simulink model "Boeing737Sample_updatedCopy"  (Simulink 8.2)
settings: Solver=ode45  StartTime=0.0  StopTime=100  RelTol=1e-3
InitFcn:
  | load('loss_coeff_mixing_junction.mat')
  | %load('defaultMSSN.mat')
  | load('SampleOutput.mat')
  | load('HydProp.mat')
  | load('HydraulicLoad.mat')
  | load('initavload.mat')
  | %load('mission_short.mat')
values from neighbouring files (symbols this model uses):
  avload =     [Benchmark_data1.mat]
  FuelBurn = [0 0 0 0 0 0 0 0 0 0 0 0 ... (18249 elements, 1x18249)]    [Benchmark_data1.mat]
undefined symbols (not defined in the file or in its folder): ailerons, B_737, elevator, F1, F2, HUGHES_TREITLER, landing_gear, PN_70147, rudder, thrust_rev
libraries: PowerFlowLib x91, simulink x19
(part 6 of 8)

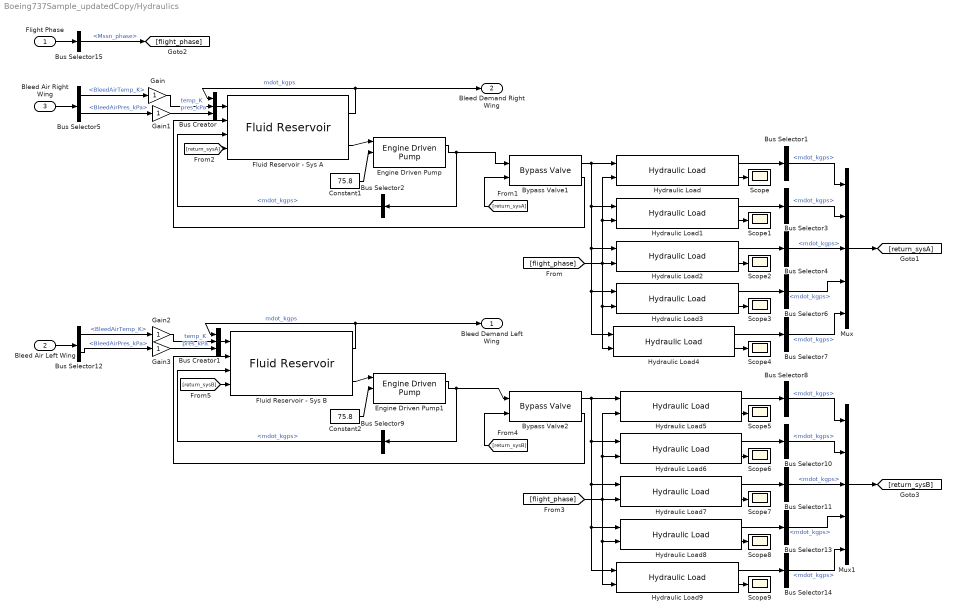
== system Boeing737Sample_updatedCopy/Hydraulics  ==
  Flight Phase : Inport
  Bleed Air Left Wing : Inport  Port=2
  Bleed Air Right Wing : Inport  Port=3
  Bus Creator : BusCreator  Inputs=3
  Bus Creator1 : BusCreator  Inputs=3
  Bus Selector{1..4,6..11,13..14} (12 alike) : BusSelector  OutputSignals=mdot_kgps
  Bus Selector12 : BusSelector  OutputSignals=Bleed.BleedAirTemp_K,Bleed.BleedAirPres_kPa
  Bus Selector15 : BusSelector  OutputSignals=Mssn_phase
  Bus Selector5 : BusSelector  OutputSignals=Bleed.BleedAirTemp_K,Bleed.BleedAirPres_kPa
  Bypass Valve1 : PowerFlowLib/Energy & Power Systems/Hydraulic/Bypass Valve
  Bypass Valve2 : PowerFlowLib/Energy & Power Systems/Hydraulic/Bypass Valve
  Constant1 : Constant  Value=75.8
  Constant2 : Constant  Value=75.8
  Engine Driven Pump : PowerFlowLib/Energy & Power Systems/Hydraulic/Engine Driven Pump  RPM=3750  disp=39  eta_mech=95  eta_v=85  nom_T=40  nom_w=393  nom_delP=20684
  Engine Driven Pump1 : PowerFlowLib/Energy & Power Systems/Hydraulic/Engine Driven Pump  RPM=3750  disp=39  eta_mech=95  eta_v=85  nom_T=40  nom_w=393  nom_delP=20684
  Fluid Reservoir - Sys A : PowerFlowLib/Energy & Power Systems/Hydraulic/Fluid Reservoir  res_vol=.25  bleed_flowrate=.05  pres_loss=1  T_init=300  P_init=1500  mass_init=30
  Fluid Reservoir - Sys B : PowerFlowLib/Energy & Power Systems/Hydraulic/Fluid Reservoir  res_vol=.25  bleed_flowrate=.05  pres_loss=1  T_init=300  P_init=1500  mass_init=30
  Gain{,1..3} (4 alike) : Gain
  Hydraulic Load : PowerFlowLib/Energy & Power Systems/Hydraulic/Hydraulic Load  fileslct=off  filename=HydraulicLoad.mat  filedir=C:\Users\mwillms4\Dropbox\School\Graduate\Research\PowerFlow Development\PowerFlow Summer 2013\PropertyTables\HydraulicLoad.mat  var_struct=HydraulicLoad  h_load=B_737 - rudder
  Hydraulic Load1 : PowerFlowLib/Energy & Power Systems/Hydraulic/Hydraulic Load  fileslct=off  filename=HydraulicLoad.mat  filedir=C:\Users\mwillms4\Dropbox\School\Graduate\Research\PowerFlow Development\PowerFlow Summer 2013\PropertyTables\HydraulicLoad.mat  var_struct=HydraulicLoad  h_load=B_737 - ailerons
  Hydraulic Load2 : PowerFlowLib/Energy & Power Systems/Hydraulic/Hydraulic Load  fileslct=off  filename=HydraulicLoad.mat  filedir=C:\Users\mwillms4\Dropbox\School\Graduate\Research\PowerFlow Development\PowerFlow Summer 2013\PropertyTables\HydraulicLoad.mat  var_struct=HydraulicLoad  h_load=B_737 - elevator
  Hydraulic Load3 : PowerFlowLib/Energy & Power Systems/Hydraulic/Hydraulic Load  fileslct=off  filename=HydraulicLoad.mat  filedir=C:\Users\mwillms4\Dropbox\School\Graduate\Research\PowerFlow Development\PowerFlow Summer 2013\PropertyTables\HydraulicLoad.mat  var_struct=HydraulicLoad  h_load=B_737 - landing_gear
  Hydraulic Load4 : PowerFlowLib/Energy & Power Systems/Hydraulic/Hydraulic Load  fileslct=off  filename=HydraulicLoad.mat  filedir=C:\Users\mwillms4\Dropbox\School\Graduate\Research\PowerFlow Development\PowerFlow Summer 2013\PropertyTables\HydraulicLoad.mat  var_struct=HydraulicLoad  h_load=B_737 - thrust_rev
  Hydraulic Load5 : PowerFlowLib/Energy & Power Systems/Hydraulic/Hydraulic Load  fileslct=off  filename=HydraulicLoad.mat  filedir=C:\Users\mwillms4\Dropbox\School\Graduate\Research\PowerFlow Development\PowerFlow Summer 2013\PropertyTables\HydraulicLoad.mat  var_struct=HydraulicLoad  h_load=B_737 - rudder
  Hydraulic Load6 : PowerFlowLib/Energy & Power Systems/Hydraulic/Hydraulic Load  fileslct=off  filename=HydraulicLoad.mat  filedir=C:\Users\mwillms4\Dropbox\School\Graduate\Research\PowerFlow Development\PowerFlow Summer 2013\PropertyTables\HydraulicLoad.mat  var_struct=HydraulicLoad  h_load=B_737 - ailerons
  Hydraulic Load7 : PowerFlowLib/Energy & Power Systems/Hydraulic/Hydraulic Load  fileslct=off  filename=HydraulicLoad.mat  filedir=C:\Users\mwillms4\Dropbox\School\Graduate\Research\PowerFlow Development\PowerFlow Summer 2013\PropertyTables\HydraulicLoad.mat  var_struct=HydraulicLoad  h_load=B_737 - elevator
  Hydraulic Load8 : PowerFlowLib/Energy & Power Systems/Hydraulic/Hydraulic Load  fileslct=off  filename=HydraulicLoad.mat  filedir=C:\Users\mwillms4\Dropbox\School\Graduate\Research\PowerFlow Development\PowerFlow Summer 2013\PropertyTables\HydraulicLoad.mat  var_struct=HydraulicLoad  h_load=B_737 - landing_gear
  Hydraulic Load9 : PowerFlowLib/Energy & Power Systems/Hydraulic/Hydraulic Load  fileslct=off  filename=HydraulicLoad.mat  filedir=C:\Users\mwillms4\Dropbox\School\Graduate\Research\PowerFlow Development\PowerFlow Summer 2013\PropertyTables\HydraulicLoad.mat  var_struct=HydraulicLoad  h_load=B_737 - thrust_rev
  Mux : Mux  Inputs=5
  Mux1 : Mux  Inputs=5
  Scope{,1..9} (10 alike) : Scope
      Scope1 settings: SaveName=ScopeData4
      Scope2 settings: YMin=0  YMax=55  SaveName=ScopeData5
      Scope3 settings: YMin=0  YMax=55
      Scope4 settings: YMin=0  YMax=55  SaveName=ScopeData2
      Scope5 settings: SaveName=ScopeData3
      Scope6 settings: SaveName=ScopeData6
      Scope7 settings: YMin=0  YMax=55  SaveName=ScopeData7
      Scope8 settings: YMin=0  YMax=55  SaveName=ScopeData8
      Scope9 settings: YMin=0  YMax=55  SaveName=ScopeData9
  Bleed Demand Left Wing : Outport
  Bleed Demand Right Wing : Outport  Port=2
  wires:
  Bus Creator/1 -> Fluid Reservoir - Sys A/1
  Bus Selector5/1 -> Gain/1  "<BleedAirTemp_K>"
  Bus Selector5/2 -> Gain1/1  "<BleedAirPres_kPa>"
  Hydraulic Load/1 -> Bus Selector1/1
  Fluid Reservoir - Sys A/2 -> Engine Driven Pump/1
  Engine Driven Pump/1 -> Bus Selector2/1, Bypass Valve1/1
  Bypass Valve1/1 -> Hydraulic Load3/1, Hydraulic Load4/1, Hydraulic Load2/1, Hydraulic Load1/1, Hydraulic Load/1
  Constant1/1 -> Engine Driven Pump/2
  Bus Selector2/1 -> Fluid Reservoir - Sys A/3  "<mdot_kgps>"
  Bypass Valve1/2 -> Fluid Reservoir - Sys A/2
  Hydraulic Load/2 -> Scope/1
  Fluid Reservoir - Sys A/1 -> Bus Creator/1, Bleed Demand Right Wing/1  "mdot_kgps"
  Hydraulic Load1/2 -> Scope1/1
  Hydraulic Load2/2 -> Scope2/1
  Hydraulic Load1/1 -> Bus Selector3/1
  Hydraulic Load2/1 -> Bus Selector4/1
  Bus Selector3/1 -> Mux/2  "<mdot_kgps>"
  Bus Selector1/1 -> Mux/1  "<mdot_kgps>"
  Bus Selector4/1 -> Mux/3  "<mdot_kgps>"
  Mux/1 -> [return_sysA]
  [return_sysA] -> Bypass Valve1/2
  [return_sysA] -> Fluid Reservoir - Sys A/4
  [flight_phase] -> Hydraulic Load/2, Hydraulic Load1/2, Hydraulic Load3/2, Hydraulic Load4/2, Hydraulic Load2/2
  Bleed Air Right Wing/1 -> Bus Selector5/1
  Hydraulic Load3/1 -> Bus Selector6/1
  Hydraulic Load4/1 -> Bus Selector7/1
  Hydraulic Load4/2 -> Scope4/1
  Hydraulic Load3/2 -> Scope3/1
  Bus Selector6/1 -> Mux/4  "<mdot_kgps>"
  Bus Selector7/1 -> Mux/5  "<mdot_kgps>"
  Bus Creator1/1 -> Fluid Reservoir - Sys B/1
  Bus Selector12/1 -> Gain2/1  "<BleedAirTemp_K>"
  Bus Selector12/2 -> Gain3/1  "<BleedAirPres_kPa>"
  Hydraulic Load5/1 -> Bus Selector8/1
  Fluid Reservoir - Sys B/2 -> Engine Driven Pump1/1
  Engine Driven Pump1/1 -> Bus Selector9/1, Bypass Valve2/1
  Bypass Valve2/1 -> Hydraulic Load9/1, Hydraulic Load8/1, Hydraulic Load7/1, Hydraulic Load6/1, Hydraulic Load5/1
  Constant2/1 -> Engine Driven Pump1/2
  Bus Selector9/1 -> Fluid Reservoir - Sys B/3  "<mdot_kgps>"
  Bypass Valve2/2 -> Fluid Reservoir - Sys B/2
  Hydraulic Load5/2 -> Scope5/1
  Fluid Reservoir - Sys B/1 -> Bus Creator1/1, Bleed Demand Left Wing/1  "mdot_kgps"
  Hydraulic Load6/2 -> Scope6/1
  Hydraulic Load7/2 -> Scope7/1
  Hydraulic Load6/1 -> Bus Selector10/1
  Hydraulic Load7/1 -> Bus Selector11/1
  Bus Selector10/1 -> Mux1/2  "<mdot_kgps>"
  Bus Selector8/1 -> Mux1/1  "<mdot_kgps>"
  Bus Selector11/1 -> Mux1/3  "<mdot_kgps>"
  Mux1/1 -> [return_sysB]
  [return_sysB] -> Bypass Valve2/2
  [return_sysB] -> Fluid Reservoir - Sys B/4
  [flight_phase] -> Hydraulic Load6/2, Hydraulic Load5/2, Hydraulic Load9/2, Hydraulic Load8/2, Hydraulic Load7/2
  Bleed Air Left Wing/1 -> Bus Selector12/1
  Hydraulic Load8/1 -> Bus Selector13/1
  Hydraulic Load9/1 -> Bus Selector14/1
  Hydraulic Load9/2 -> Scope9/1
  Hydraulic Load8/2 -> Scope8/1
  Bus Selector13/1 -> Mux1/4  "<mdot_kgps>"
  Bus Selector14/1 -> Mux1/5  "<mdot_kgps>"
  Flight Phase/1 -> Bus Selector15/1
  Bus Selector15/1 -> [flight_phase]  "<Mssn_phase>"
  Gain/1 -> Bus Creator/2  "temp_K"
  Gain1/1 -> Bus Creator/3  "pres_kPa"
  Gain2/1 -> Bus Creator1/2  "temp_K"
  Gain3/1 -> Bus Creator1/3  "pres_kPa"

== system Boeing737Sample_updatedCopy/PowerFlow Data Manager ==
  Data : Outport

== system Boeing737Sample_updatedCopy/ECS & FOS /Distributor valve ==
  Flow from Right Pack : Inport
  "Distribution ratio, R" : Inport  Port=2
  Bus Creator : BusCreator  Inputs=3
  Bus Creator1 : BusCreator  Inputs=3
  Bus Selector1 : BusSelector  OutputSignals=mdot_kgps,temp_K,pres_kPa
  M(1-R) : Sum  Inputs=+-
  Product : Product
  To cargo : Outport
  To Mix Junction : Outport  Port=2
  wires:
  Flow from Right Pack/1 -> Bus Selector1/1
  Bus Selector1/1 -> M(1-R)/1, Product/1  "<mdot_kgps>"
  "Distribution ratio, R"/1 -> Product/2
  Product/1 -> Bus Creator1/1, M(1-R)/2  "mdot_kgps"
  M(1-R)/1 -> Bus Creator/1  "mdot_kgps"
  Bus Creator/1 -> To Mix Junction/1
  Bus Creator1/1 -> To cargo/1
  Bus Selector1/2 -> Bus Creator/2, Bus Creator1/2  "<temp_K>"
  Bus Selector1/3 -> Bus Creator/3, Bus Creator1/3  "<pres_kPa>"

== system Boeing737Sample_updatedCopy/ECS & FOS /FOHX Left Wing ==
  Flow1In : Inport
  Flow2In : Inport  Port=2
  Bias : Bias  Bias=-35
  Bias1 : Bias  Bias=-35
  Bus Creator1 : BusCreator  Inputs=6
  Bus Creator2 : BusCreator
  Bus Creator3 : BusCreator
  Bus Selector1 : BusSelector  OutputSignals=h2_out,T2_out
  Bus Selector2 : BusSelector  OutputSignals=mdot_kgps,pres_kPa,temp_K
  Bus Selector3 : BusSelector  OutputSignals=mdot2_in
  Bus Selector5 : BusSelector  OutputSignals=mdot_kgps,temp_K,pres_kPa
  Bus Selector7 : BusSelector  OutputSignals=h1_out,T1_out
  Bus Selector9 : BusSelector  OutputSignals=mdot1_in
  Gain{,1..13} (14 alike) : Gain
  HX_Calcs : Subsystem
  F1out : Outport
  F2out : Outport  Port=2
  wires:
  Bias1/1 -> Gain11/1
  Bias/1 -> Bus Creator2/1  "pres_kPa"
  Gain13/1 -> Bias/1  "pres_kPa"
  Gain11/1 -> Bus Creator3/1  "pres_kPa"
  Gain8/1 -> Bus Creator2/2  "mdot_kgps"
  Bus Selector3/1 -> Gain8/1  "<mdot2_in>"
  Gain5/1 -> Bus Creator2/3  "h_kJ/kg"
  Gain7/1 -> Bus Creator2/4  "temp_K"
  [Outputs] -> Bus Selector1/1
  Bus Selector1/1 -> Gain5/1  "<h2_out>"
  Bus Selector1/2 -> Gain7/1  "<T2_out>"
  Gain3/1 -> Gain13/1, Bus Creator1/6  "P2_in"
  Bus Selector5/3 -> Gain3/1  "<pres_kPa>"
  Gain/1 -> Bus Creator1/1  "mdot1_in"
  Gain1/1 -> Bias1/1, Bus Creator1/2  "P1_in"
  Gain2/1 -> Bus Creator1/3  "T1_in"
  Gain4/1 -> Bus Creator1/4  "mdot2_in"
  Gain6/1 -> Bus Creator1/5  "T2_in"
  HX_Calcs/1(Out) -> [Outputs]
  Flow1In/1 -> Bus Selector2/1
  Bus Creator1/1 -> Bus Selector3/1, Bus Selector9/1, HX_Calcs/1(Inputs)
  Bus Selector2/1 -> Gain/1  "<mdot_kgps>"
  Bus Selector2/2 -> Gain1/1  "<pres_kPa>"
  Bus Selector2/3 -> Gain2/1  "<temp_K>"
  Flow2In/1 -> Bus Selector5/1
  Bus Selector5/2 -> Gain6/1  "<temp_K>"
  Bus Selector5/1 -> Gain4/1  "<mdot_kgps>"
  Bus Creator2/1 -> F2out/1
  Bus Creator3/1 -> F1out/1
  Gain12/1 -> Bus Creator3/2  "mdot_kgps"
  Gain10/1 -> Bus Creator3/3  "h_kJ/kg"
  Gain9/1 -> Bus Creator3/4  "temp_K"
  [Outputs] -> Bus Selector7/1
  Bus Selector9/1 -> Gain12/1  "<mdot1_in>"
  Bus Selector7/1 -> Gain10/1  "<h1_out>"
  Bus Selector7/2 -> Gain9/1  "<T1_out>"

== system Boeing737Sample_updatedCopy/ECS & FOS /FOHX Right Wing ==
  Flow1In : Inport
  Flow2In : Inport  Port=2
  Bias : Bias  Bias=-35
  Bias1 : Bias  Bias=-35
  Bus Creator1 : BusCreator  Inputs=6
  Bus Creator2 : BusCreator
  Bus Creator3 : BusCreator
  Bus Selector1 : BusSelector  OutputSignals=h2_out,T2_out
  Bus Selector2 : BusSelector  OutputSignals=mdot_kgps,pres_kPa,temp_K
  Bus Selector3 : BusSelector  OutputSignals=mdot2_in
  Bus Selector5 : BusSelector  OutputSignals=mdot_kgps,temp_K,pres_kPa
  Bus Selector7 : BusSelector  OutputSignals=h1_out,T1_out
  Bus Selector9 : BusSelector  OutputSignals=mdot1_in
  Gain{,1..13} (14 alike) : Gain
  HX_Calcs : Subsystem
  F1out : Outport
  F2out : Outport  Port=2
  wires:
  Bus Selector7/2 -> Gain9/1  "<T1_out>"
  Bus Selector7/1 -> Gain10/1  "<h1_out>"
  Bus Selector9/1 -> Gain12/1  "<mdot1_in>"
  [Outputs] -> Bus Selector7/1
  Gain9/1 -> Bus Creator3/4  "temp_K"
  Gain10/1 -> Bus Creator3/3  "h_kJ/kg"
  Gain12/1 -> Bus Creator3/2  "mdot_kgps"
  Bus Creator3/1 -> F1out/1
  Bus Creator2/1 -> F2out/1
  Bus Selector5/1 -> Gain4/1  "<mdot_kgps>"
  Bus Selector5/2 -> Gain6/1  "<temp_K>"
  Flow2In/1 -> Bus Selector5/1
  Bus Selector2/3 -> Gain2/1  "<temp_K>"
  Bus Selector2/2 -> Gain1/1  "<pres_kPa>"
  Bus Selector2/1 -> Gain/1  "<mdot_kgps>"
  Bus Creator1/1 -> HX_Calcs/1(Inputs), Bus Selector9/1, Bus Selector3/1
  Flow1In/1 -> Bus Selector2/1
  HX_Calcs/1(Out) -> [Outputs]
  Gain6/1 -> Bus Creator1/5  "T2_in"
  Gain4/1 -> Bus Creator1/4  "mdot2_in"
  Gain2/1 -> Bus Creator1/3  "T1_in"
  Gain1/1 -> Bus Creator1/2, Bias1/1  "P1_in"
  Gain/1 -> Bus Creator1/1  "mdot1_in"
  Bus Selector5/3 -> Gain3/1  "<pres_kPa>"
  Gain3/1 -> Bus Creator1/6, Gain13/1  "P2_in"
  Bus Selector1/2 -> Gain7/1  "<T2_out>"
  Bus Selector1/1 -> Gain5/1  "<h2_out>"
  [Outputs] -> Bus Selector1/1
  Gain7/1 -> Bus Creator2/4  "temp_K"
  Gain5/1 -> Bus Creator2/3  "h_kJ/kg"
  Bus Selector3/1 -> Gain8/1  "<mdot2_in>"
  Gain8/1 -> Bus Creator2/2  "mdot_kgps"
  Gain11/1 -> Bus Creator3/1  "pres_kPa"
  Gain13/1 -> Bias/1  "pres_kPa"
  Bias/1 -> Bus Creator2/1  "pres_kPa"
  Bias1/1 -> Gain11/1

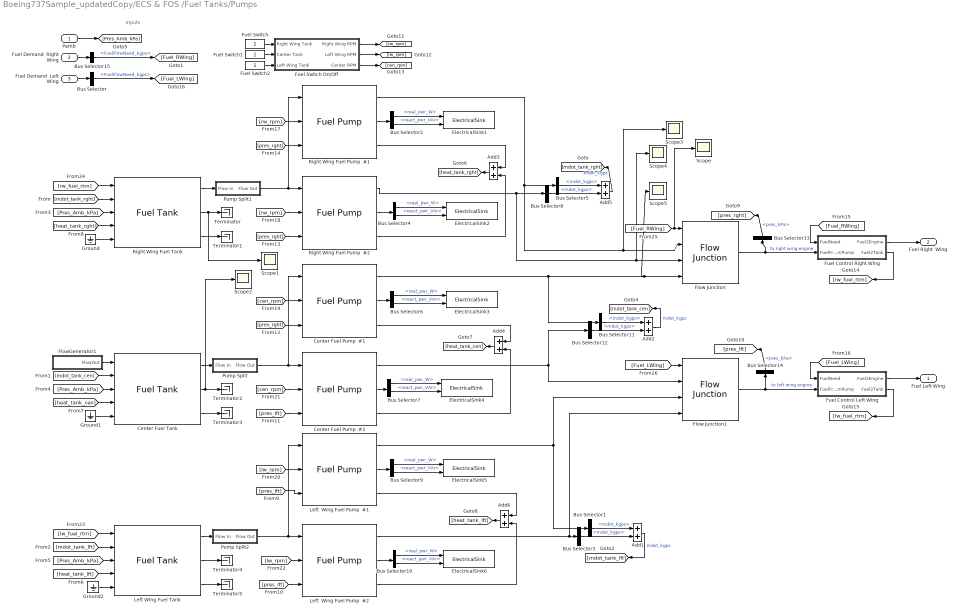
== system Boeing737Sample_updatedCopy/ECS & FOS /Fuel Tanks/Pumps ==
  note: Inputs
  Pamb : Inport
  Fuel Demand  Right Wing : Inport  Port=2
  Fuel Demand  Left Wing : Inport  Port=3
  Add{1..6} (6 alike) : Sum
  Bus Selector : BusSelector  OutputSignals=Fuel.FuelFlowNeed_kgps
  Bus Selector{1,3,5,8,11..12} (6 alike) : BusSelector  OutputSignals=mdot_kgps
  Bus Selector{2,4,6..7,9..10} (6 alike) : BusSelector  OutputSignals=real_pwr_W,react_pwr_VAr
  Bus Selector13 : BusSelector  OutputSignals=pres_kPa
  Bus Selector14 : BusSelector  OutputSignals=pres_kPa
  Bus Selector15 : BusSelector  OutputSignals=Fuel.FuelFlowNeed_kgps
  Center Fuel Pump  #1 : PowerFlowLib/Energy & Power Systems/Thermal/Fuel/Fuel Pump  maptype=Pressure (kPa) vs. Vol. Flow Rate (m³/hr)  map=B737_AC_fuel1  map_load=off  SG=0.82  pump_eff=.75  heat_out=off  AC_pwr=on  pf=1  mech_pwr=off
  Center Fuel Pump  #2 : PowerFlowLib/Energy & Power Systems/Thermal/Fuel/Fuel Pump  maptype=Pressure (kPa) vs. Vol. Flow Rate (m³/hr)  map=B737_AC_fuel1  map_load=off  SG=0.82  pump_eff=.75  heat_out=off  AC_pwr=on  pf=1  mech_pwr=off
  Center Fuel Tank : PowerFlowLib/Energy & Power Systems/Thermal/Fuel/Fuel Tank  fileslct=off  filename=fueltank_area.m  filedir=C:\Users\mwillms4\Documents\My Box Files\Graduate\Research\PowerFlow Development\PowerFlow Fall 2013\SupportFunctions\fueltank_area.m  tank_loc=Center Tank  areaprompt2=off  max_vol=3.2  m_init=2500  fld_Tint=0  ull_Tint=30  Pover=100  HTC_fg=14.2  wallHXF=off  wetHTC=14.2  dryHTC=14.2  Qinternal=0
  ElectricalSink1 : PowerFlowLib/Support Functions//Tools/ElectricalSink  Tag=Flow  Description=TwoPhase  load_loc=RightWing  ACDC_load=AC  units=Watts  unq_id=9219
  ElectricalSink2 : PowerFlowLib/Support Functions//Tools/ElectricalSink  Tag=Flow  Description=TwoPhase  load_loc=RightWing  ACDC_load=AC  units=Watts  unq_id=5921
  ElectricalSink3 : PowerFlowLib/Support Functions//Tools/ElectricalSink  Tag=Flow  Description=TwoPhase  load_loc=RightWing  ACDC_load=AC  units=Watts  unq_id=9683
  ElectricalSink4 : PowerFlowLib/Support Functions//Tools/ElectricalSink  Tag=Flow  Description=TwoPhase  load_loc=LeftWing  ACDC_load=AC  units=Watts  unq_id=2143
  ElectricalSink5 : PowerFlowLib/Support Functions//Tools/ElectricalSink  Tag=Flow  Description=TwoPhase  load_loc=LeftWing  ACDC_load=AC  units=Watts  unq_id=2418
  ElectricalSink6 : PowerFlowLib/Support Functions//Tools/ElectricalSink  Tag=Flow  Description=TwoPhase  load_loc=LeftWing  ACDC_load=AC  units=Watts  unq_id=9734
  Flow Junction : PowerFlowLib/Energy & Power Systems/Thermal/Fuel/Flow Junction  Description=TwoPhase  V=.05  Bm=10^5  initPres=6000  initTemp=30
  Flow Junction1 : PowerFlowLib/Energy & Power Systems/Thermal/Fuel/Flow Junction  Description=TwoPhase  V=.05  Bm=10^5  initPres=6000  initTemp=30
  FlowGenerator1 : Subsystem  Tag=Flow  Description=TwoPhase  mask{fld_type1=null, flowrate=0, flowtemp=0, flowpres=00, flowenthalpy=0}
      mask prompts: fld_type1 "Fluid Type"; flowrate "Fluid Flow Rate (kg/s)"; flowtemp "Fluid Flow Temperature (C)"; flowpres "Fluid Flow Pressure (kPa)"; flowenthalpy "Fluid Flow Enthalpy (kJ/kg)"
      mask TypeOptions fld_type1: null
      mask Display: text(.5,.5,'Flow Source','horizontalAlignment','center','texmode','on')
  Fuel Control Left Wing : Subsystem
      mask Display:
      | port_label('input',1,'{\bf Fuel Need}','TexMode','on')
      | port_label('input',2,'{\bf Fuel In}','TexMode','on')
      | 
      | 
      | port_label('output',1,'{\bf Fuel to Eng.}','TexMode','on')
      | port_label('output',2,'{\bf Fuel Return}','TexMode','on')
  "Fuel Control Right Wing " : Subsystem
      mask Display:
      | port_label('input',1,'{\bf Fuel Need}','TexMode','on')
      | port_label('input',2,'{\bf Fuel In}','TexMode','on')
      | 
      | 
      | port_label('output',1,'{\bf Fuel to Eng.}','TexMode','on')
      | port_label('output',2,'{\bf Fuel Return}','TexMode','on')
  Fuel Switch : Constant
  Fuel Switch On/Off : Subsystem
  Fuel Switch1 : Constant
  Fuel Switch2 : Constant
  Ground : Ground
  Ground1 : Ground
  Ground2 : Ground
  Left  Wing Fuel Pump  #1 : PowerFlowLib/Energy & Power Systems/Thermal/Fuel/Fuel Pump  maptype=Pressure (kPa) vs. Vol. Flow Rate (m³/hr)  map=B737_AC_fuel1  map_load=off  SG=0.82  pump_eff=.75  heat_out=off  AC_pwr=on  pf=1  mech_pwr=off
  Left  Wing Fuel Pump  #2 : PowerFlowLib/Energy & Power Systems/Thermal/Fuel/Fuel Pump  maptype=Pressure (kPa) vs. Vol. Flow Rate (m³/hr)  map=B737_AC_fuel1  map_load=off  SG=0.82  pump_eff=.75  heat_out=off  AC_pwr=on  pf=1  mech_pwr=off
  Left Wing Fuel Tank : PowerFlowLib/Energy & Power Systems/Thermal/Fuel/Fuel Tank  fileslct=off  filename=fueltank_area.m  filedir=C:\Users\mwillms4\Documents\My Box Files\Graduate\Research\PowerFlow Development\PowerFlow Fall 2013\SupportFunctions\fueltank_area.m  tank_loc=Left Wing Tank  areaprompt2=off  max_vol=3.2  m_init=2500  fld_Tint=0  ull_Tint=30  Pover=100  HTC_fg=14.2  wallHXF=off  wetHTC=14.2  dryHTC=14.2  Qinternal=0
  Pump Split : Subsystem
  Pump Split1 : Subsystem
  Pump Split2 : Subsystem
  Right Wing Fuel Pump  #1 : PowerFlowLib/Energy & Power Systems/Thermal/Fuel/Fuel Pump  maptype=Pressure (kPa) vs. Vol. Flow Rate (m³/hr)  map=B737_AC_fuel1  map_load=off  SG=0.82  pump_eff=.75  heat_out=off  AC_pwr=on  pf=1  mech_pwr=off
  Right Wing Fuel Pump  #2 : PowerFlowLib/Energy & Power Systems/Thermal/Fuel/Fuel Pump  maptype=Pressure (kPa) vs. Vol. Flow Rate (m³/hr)  map=B737_AC_fuel1  map_load=off  SG=0.82  pump_eff=.75  heat_out=off  AC_pwr=on  pf=1  mech_pwr=off
  Right Wing Fuel Tank : PowerFlowLib/Energy & Power Systems/Thermal/Fuel/Fuel Tank  fileslct=off  filename=fueltank_area.m  filedir=C:\Users\mwillms4\Documents\My Box Files\Graduate\Research\PowerFlow Development\PowerFlow Fall 2013\SupportFunctions\fueltank_area.m  tank_loc=Right Wing Tank  areaprompt2=off  max_vol=3.2  m_init=2500  fld_Tint=0  ull_Tint=30  Pover=100  HTC_fg=14.2  wallHXF=off  wetHTC=14.2  dryHTC=14.2  Qinternal=0
  Scope{,1..5} (6 alike) : Scope
      Scope settings: SaveName=ScopeData21
      Scope1 settings: YMin=2498.9  YMax=2498.9  SaveName=ScopeData23
      Scope2 settings: SaveName=ScopeData25
      Scope3 settings: SaveName=ScopeData27
      Scope4 settings: SaveName=ScopeData28
      Scope5 settings: SaveName=ScopeData29
  Terminator{,1..5} (6 alike) : Terminator
  Fuel Left Wing : Outport
  Fuel Right  Wing : Outport  Port=2
  wires:
  Pamb/1 -> [Pres_Amb_kPa]
  Fuel Switch/1 -> Fuel Switch On/Off/1(Right Wing Tank)
  Fuel Switch1/1 -> Fuel Switch On/Off/2(Center Tank)
  Fuel Switch2/1 -> Fuel Switch On/Off/3(Left Wing Tank)
  Fuel Switch On/Off/1(Right Wing RPM) -> [rw_rpm]
  Fuel Switch On/Off/2(Left Wing RPM) -> [lw_rpm]
  Fuel Switch On/Off/3(Center RPM) -> [cen_rpm]
  Left  Wing Fuel Pump  #2/1 -> Bus Selector3/1, Flow Junction1/4
  [lw_fuel_rtrn] -> Left Wing Fuel Tank/1
  Left  Wing Fuel Pump  #2/2 -> Bus Selector10/1
  Left  Wing Fuel Pump  #1/1 -> Bus Selector1/1, Flow Junction1/3
  Left  Wing Fuel Pump  #1/2 -> Bus Selector9/1
  Center Fuel Pump  #2/1 -> Bus Selector12/1, Flow Junction1/2
  FlowGenerator1/1(FlowOut) -> Center Fuel Tank/1
  Center Fuel Pump  #2/2 -> Bus Selector7/1
  Flow Junction1/1 -> Bus Selector14/1, Fuel Control Left Wing/2(FuelFromPump)  "to left wing engine"
  Center Fuel Pump  #1/1 -> Bus Selector11/1, Flow Junction/4, Scope5/1
  Center Fuel Pump  #1/2 -> Bus Selector6/1
  Flow Junction/1 -> Bus Selector13/1, "Fuel Control Right Wing "/2(FuelFromPump)  "to right wing engine"
  Center Fuel Tank/1 -> Pump Split/1(Flow In)
  Right Wing Fuel Pump  #2/1 -> Bus Selector8/1, Flow Junction/3, Scope4/1
  [rw_fuel_rtrn] -> Right Wing Fuel Tank/1
  Right Wing Fuel Pump  #2/2 -> Bus Selector4/1
  Right Wing Fuel Pump  #1/1 -> Bus Selector5/1, Flow Junction/2, Scope3/1
  [rw_rpm] -> Right Wing Fuel Pump  #1/2
  Right Wing Fuel Tank/1 -> Pump Split1/1(Flow In)
  Pump Split1/1(Flow Out) -> Right Wing Fuel Pump  #1/1, Right Wing Fuel Pump  #2/1
  Bus Selector8/1 -> Add5/2  "<mdot_kgps>"
  [mdot_tank_rght] -> Right Wing Fuel Tank/2
  [mdot_tank_cen] -> Center Fuel Tank/2
  [mdot_tank_lft] -> Left Wing Fuel Tank/2
  Pump Split/1(Flow Out) -> Center Fuel Pump  #1/1, Center Fuel Pump  #2/1
  Left Wing Fuel Tank/1 -> Pump Split2/1(Flow In)
  Bus Selector5/1 -> Add5/1  "<mdot_kgps>"
  Add5/1 -> [mdot_tank_rght]  "mdot_kgps"
  Bus Selector3/1 -> Add1/2  "<mdot_kgps>"
  Bus Selector1/1 -> Add1/1  "<mdot_kgps>"
  Add1/1 -> [mdot_tank_lft]  "mdot_kgps"
  Bus Selector12/1 -> Add2/2  "<mdot_kgps>"
  Bus Selector11/1 -> Add2/1  "<mdot_kgps>"
  Add2/1 -> [mdot_tank_cen]  "mdot_kgps"
  [Pres_Amb_kPa] -> Right Wing Fuel Tank/3
  [Pres_Amb_kPa] -> Center Fuel Tank/3
  [Pres_Amb_kPa] -> Left Wing Fuel Tank/3
  Add6/1 -> [heat_tank_lft]
  [heat_tank_lft] -> Left Wing Fuel Tank/4
  [heat_tank_cen] -> Center Fuel Tank/4
  [heat_tank_rght] -> Right Wing Fuel Tank/4
  Bus Selector13/1 -> [pres_rght]  "<pres_kPa>"
  [rw_rpm] -> Right Wing Fuel Pump  #2/2
  [cen_rpm] -> Center Fuel Pump  #1/2
  [cen_rpm] -> Center Fuel Pump  #2/2
  [lw_rpm] -> Left  Wing Fuel Pump  #1/2
  [lw_rpm] -> Left  Wing Fuel Pump  #2/2
  Bus Selector14/1 -> [pres_lft]  "<pres_kPa>"
  [pres_lft] -> Left  Wing Fuel Pump  #1/3
  [pres_lft] -> Left  Wing Fuel Pump  #2/3
  [pres_lft] -> Center Fuel Pump  #2/3
  [pres_rght] -> Center Fuel Pump  #1/3
  [pres_rght] -> Right Wing Fuel Pump  #2/3
  [pres_rght] -> Right Wing Fuel Pump  #1/3
  [Fuel_LWing] -> Flow Junction1/1
  [Fuel_RWing] -> Flow Junction/1, Scope/1
  Right Wing Fuel Tank/2 -> Terminator/1, Scope1/1
  Right Wing Fuel Tank/3 -> Terminator1/1
  Center Fuel Tank/2 -> Terminator2/1, Scope2/1
  Center Fuel Tank/3 -> Terminator3/1
  Left Wing Fuel Tank/2 -> Terminator4/1
  Left Wing Fuel Tank/3 -> Terminator5/1
  Ground/1 -> Right Wing Fuel Tank/5
  Ground1/1 -> Center Fuel Tank/5
  Ground2/1 -> Left Wing Fuel Tank/5
  Fuel Demand  Left Wing/1 -> Bus Selector/1
  [Fuel_RWing] -> "Fuel Control Right Wing "/1(FuelNeed)
  [Fuel_LWing] -> Fuel Control Left Wing/1(FuelNeed)
  Fuel Control Left Wing/2(Fuel2Tank) -> [lw_fuel_rtrn]
  "Fuel Control Right Wing "/2(Fuel2Tank) -> [rw_fuel_rtrn]
  "Fuel Control Right Wing "/1(Fuel2Engine) -> Fuel Right  Wing/1
  Fuel Control Left Wing/1(Fuel2Engine) -> Fuel Left Wing/1
  Pump Split2/1(Flow Out) -> Left  Wing Fuel Pump  #1/1, Left  Wing Fuel Pump  #2/1
  Bus Selector/1 -> [Fuel_LWing]  "<FuelFlowNeed_kgps>"
  Fuel Demand  Right Wing/1 -> Bus Selector15/1
  Bus Selector15/1 -> [Fuel_RWing]  "<FuelFlowNeed_kgps>"
  Bus Selector2/1 -> ElectricalSink1/1  "<real_pwr_W>"
  Add4/1 -> [heat_tank_cen]
  Add3/1 -> [heat_tank_rght]
  Right Wing Fuel Pump  #1/2 -> Bus Selector2/1
  Bus Selector2/2 -> ElectricalSink1/2  "<react_pwr_VAr>"
  Bus Selector4/1 -> ElectricalSink2/1  "<real_pwr_W>"
  Bus Selector4/2 -> ElectricalSink2/2  "<react_pwr_VAr>"
  Bus Selector6/1 -> ElectricalSink3/1  "<real_pwr_W>"
  Bus Selector6/2 -> ElectricalSink3/2  "<react_pwr_VAr>"
  Bus Selector7/1 -> ElectricalSink4/1  "<real_pwr_W>"
  Bus Selector7/2 -> ElectricalSink4/2  "<react_pwr_VAr>"
  Bus Selector9/1 -> ElectricalSink5/1  "<real_pwr_W>"
  Bus Selector9/2 -> ElectricalSink5/2  "<react_pwr_VAr>"
  Bus Selector10/1 -> ElectricalSink6/1  "<real_pwr_W>"
  Bus Selector10/2 -> ElectricalSink6/2  "<react_pwr_VAr>"
  Right Wing Fuel Pump  #1/3 -> Add3/1
  Right Wing Fuel Pump  #2/3 -> Add3/2
  Center Fuel Pump  #1/3 -> Add4/1
  Center Fuel Pump  #2/3 -> Add4/2
  Left  Wing Fuel Pump  #1/3 -> Add6/1
  Left  Wing Fuel Pump  #2/3 -> Add6/2

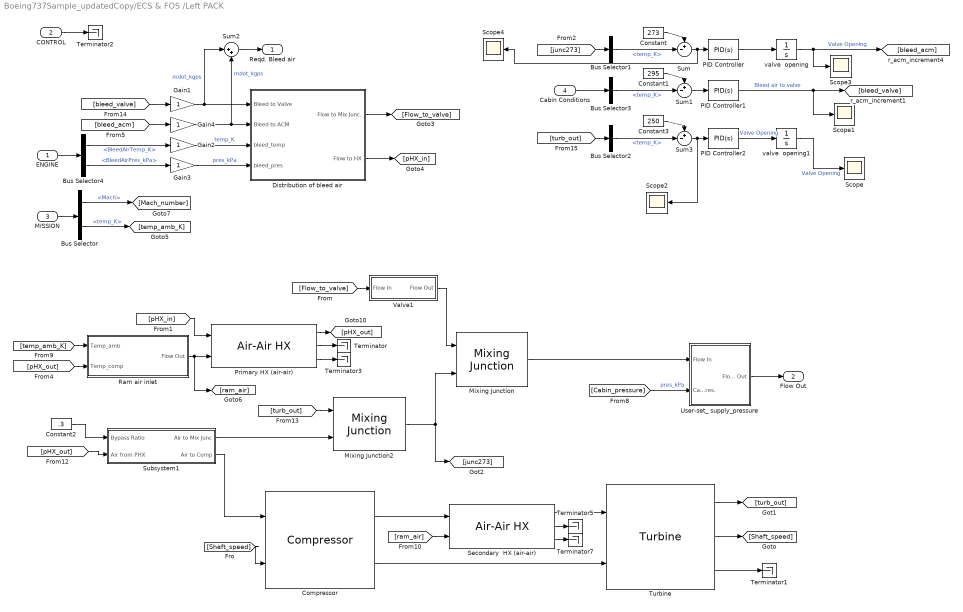
== system Boeing737Sample_updatedCopy/ECS & FOS /Left PACK ==
  ENGINE : Inport
  CONTROL : Inport  Port=2
  MISSION : Inport  Port=3
  Cabin Conditions : Inport  Port=4
  Bus Selector : BusSelector  OutputSignals=Flight parameters.Mach,Flight parameters.temp_K
  Bus Selector1 : BusSelector  OutputSignals=temp_K
  Bus Selector2 : BusSelector  OutputSignals=temp_K
  Bus Selector3 : BusSelector  OutputSignals=temp_K
  Bus Selector4 : BusSelector  OutputSignals=Bleed.BleedAirTemp_K,Bleed.BleedAirPres_kPa
  Compressor : PowerFlowLib/Energy & Power Systems/Thermal/ECS/Compressor
  Constant : Constant  Value=273
  Constant1 : Constant  Value=295
  Constant2 : Constant  Value=.3
  Constant3 : Constant  Value=250
  Distribution of bleed air : Subsystem
      mask Display:
      | port_label('input',1,'{ \bfBleed air to valve [kg/s]}','texmode','on')
      | port_label('input',2,'{ \bfBleed air to ACM [kg/s]}','texmode','on')
      | port_label('input',3,'{ \bfBleed temp. (K)}','texmode','on');
      | port_label('input',4,'{ \bfBleed pressure. (kPa)}','texmode','on')
      | 
      | 
      | 
      | port_label('output',1,'{\bfFlow to Mix Junc. }','texmode','on')
      | port_label('output',2,'{\bfFlow to ACM }','texmode','on')
  Gain{1..4} (4 alike) : Gain
  Mixing Junction : PowerFlowLib/Energy & Power Systems/Thermal/ECS/Mixing Junction  d_in_1=0.1  d_in_2=0.1  d_out=0.2
  Mixing Junction2 : PowerFlowLib/Energy & Power Systems/Thermal/ECS/Mixing Junction  d_in_1=0.1  d_in_2=0.1  d_out=0.2
  PID Controller : simulink/Continuous/PID Controller  Controller=PID  TimeDomain=Continuous-time  SampleTime=1  IntegratorMethod=Forward Euler  FilterMethod=Forward Euler  Form=Parallel  P=.01  I=0  D=0  N=100  InitialConditionSource=internal  InitialConditionForIntegrator=0  InitialConditionForFilter=0  ExternalReset=none  LimitOutput=off  UpperSaturationLimit=inf  LowerSaturationLimit=-inf  LinearizeAsGain=off  AntiWindupMode=none  Kb=1  TrackingMode=off  Kt=1  PParamMin=[]  PParamMax=[]  IParamMin=[]  IParamMax=[]  DParamMin=[]  DParamMax=[]  NParamMin=[]  NParamMax=[]  KbParamMin=[]  KbParamMax=[]  KtParamMin=[]  KtParamMax=[]  POutMin=[]  POutMax=[]  IOutMin=[]  IOutMax=[]  DOutMin=[]  DOutMax=[]  NOutMin=[]  NOutMax=[]  KbOutMin=[]  KbOutMax=[]  KtOutMin=[]  KtOutMax=[]  IntegratorOutMin=[]  IntegratorOutMax=[]  FilterOutMin=[]  FilterOutMax=[]  SumOutMin=[]  SumOutMax=[]  SumI1OutMin=[]  SumI1OutMax=[]  SumI2OutMin=[]  SumI2OutMax=[]  SumI3OutMin=[]  SumI3OutMax=[]  SumDOutMin=[]  SumDOutMax=[]  SaturationOutMin=[]  SaturationOutMax=[]  IntegratorContinuousStateAttributes=''  IntegratorStateMustResolveToSignalObject=off  IntegratorRTWStateStorageClass=Auto  FilterContinuousStateAttributes=''  FilterStateMustResolveToSignalObject=off  FilterRTWStateStorageClass=Auto
  PID Controller1 : simulink/Continuous/PID Controller  Controller=PID  TimeDomain=Continuous-time  SampleTime=1  IntegratorMethod=Forward Euler  FilterMethod=Forward Euler  Form=Parallel  P=.2  I=.01  D=0  N=100  InitialConditionSource=internal  InitialConditionForIntegrator=0  InitialConditionForFilter=0  ExternalReset=none  LimitOutput=on  UpperSaturationLimit=2  LowerSaturationLimit=.05  LinearizeAsGain=off  AntiWindupMode=none  Kb=1  TrackingMode=off  Kt=1  PParamMin=[]  PParamMax=[]  IParamMin=[]  IParamMax=[]  DParamMin=[]  DParamMax=[]  NParamMin=[]  NParamMax=[]  KbParamMin=[]  KbParamMax=[]  KtParamMin=[]  KtParamMax=[]  POutMin=[]  POutMax=[]  IOutMin=[]  IOutMax=[]  DOutMin=[]  DOutMax=[]  NOutMin=[]  NOutMax=[]  KbOutMin=[]  KbOutMax=[]  KtOutMin=[]  KtOutMax=[]  IntegratorOutMin=[]  IntegratorOutMax=[]  FilterOutMin=[]  FilterOutMax=[]  SumOutMin=[]  SumOutMax=[]  SumI1OutMin=[]  SumI1OutMax=[]  SumI2OutMin=[]  SumI2OutMax=[]  SumI3OutMin=[]  SumI3OutMax=[]  SumDOutMin=[]  SumDOutMax=[]  SaturationOutMin=[]  SaturationOutMax=[]  IntegratorContinuousStateAttributes=''  IntegratorStateMustResolveToSignalObject=off  IntegratorRTWStateStorageClass=Auto  FilterContinuousStateAttributes=''  FilterStateMustResolveToSignalObject=off  FilterRTWStateStorageClass=Auto
  PID Controller2 : simulink/Continuous/PID Controller  Controller=PID  TimeDomain=Continuous-time  SampleTime=1  IntegratorMethod=Forward Euler  FilterMethod=Forward Euler  Form=Parallel  P=0.01  I=0  D=0  N=100  InitialConditionSource=internal  InitialConditionForIntegrator=0  InitialConditionForFilter=0  ExternalReset=none  LimitOutput=off  UpperSaturationLimit=inf  LowerSaturationLimit=0  LinearizeAsGain=off  AntiWindupMode=none  Kb=1  TrackingMode=off  Kt=1  PParamMin=[]  PParamMax=[]  IParamMin=[]  IParamMax=[]  DParamMin=[]  DParamMax=[]  NParamMin=[]  NParamMax=[]  KbParamMin=[]  KbParamMax=[]  KtParamMin=[]  KtParamMax=[]  POutMin=[]  POutMax=[]  IOutMin=[]  IOutMax=[]  DOutMin=[]  DOutMax=[]  NOutMin=[]  NOutMax=[]  KbOutMin=[]  KbOutMax=[]  KtOutMin=[]  KtOutMax=[]  IntegratorOutMin=[]  IntegratorOutMax=[]  FilterOutMin=[]  FilterOutMax=[]  SumOutMin=[]  SumOutMax=[]  SumI1OutMin=[]  SumI1OutMax=[]  SumI2OutMin=[]  SumI2OutMax=[]  SumI3OutMin=[]  SumI3OutMax=[]  SumDOutMin=[]  SumDOutMax=[]  SaturationOutMin=[]  SaturationOutMax=[]  IntegratorContinuousStateAttributes=''  IntegratorStateMustResolveToSignalObject=off  IntegratorRTWStateStorageClass=Auto  FilterContinuousStateAttributes=''  FilterStateMustResolveToSignalObject=off  FilterRTWStateStorageClass=Auto
  Primary HX (air-air) : PowerFlowLib/Energy & Power Systems/Thermal/ECS/Air-Air HX  L_hx=0.2  W_hx=0.2  H_hx=0.2  t_p=0.0008  K_p=167  cp_hx=883  m_cm=16  l_fin=.005  t_fin=0.0002  s_fin=0.0015  h_fin=0.0095  K_n=167  eta_f=0.8  T_cm_0=50
  Ram air inlet : Subsystem  mask{ram_air=.5, T_35=273}
      mask prompts: ram_air "Ram air mass flow rate"; T_35 "Temperature control for 35F valve"
      mask Display:
      | port_label('input',1,'{ \bf Ambient Temp.}','texmode','on')
      | port_label('input',2,'{ \bf Comp. Face Temp.}','texmode','on');
      | 
      | port_label('output',1,'{\bf Flow Out}','texmode','on')
  Scope{,1..4} (5 alike) : Scope
      Scope settings: YMin=0  YMax=1  SaveName=ScopeData32  SampleInput=on  SampleTime=1
      Scope1 settings: SaveName=ScopeData33  SampleInput=on  SampleTime=1
      Scope2 settings: YMin=-0.0534  YMax=-0.0529  SaveName=ScopeData34  SampleInput=on  SampleTime=1
      Scope3 settings: YMin=0.28294  YMax=0.28294  SaveName=ScopeData35  SampleInput=on  SampleTime=1
      Scope4 settings: TimeRange=1500  YMin=2.8421709427e-013  YMax=2.8421709434e-013  SaveName=ScopeData37  SampleInput=on  SampleTime=1
  Secondary  HX (air-air) : PowerFlowLib/Energy & Power Systems/Thermal/ECS/Air-Air HX  L_hx=0.2  W_hx=0.2  H_hx=0.2  t_p=0.0008  K_p=167  cp_hx=883  m_cm=16  l_fin=.005  t_fin=0.0002  s_fin=0.0015  h_fin=0.0095  K_n=167  eta_f=0.8  T_cm_0=25
  Subsystem1 : Subsystem
  Sum : Sum  Inputs=+-|
  Sum1 : Sum  Inputs=+-|
  Sum2 : Sum  Inputs=|++
  Sum3 : Sum  Inputs=+-|
  Terminator{,1..3,5,7} (6 alike) : Terminator
  Turbine : PowerFlowLib/Energy & Power Systems/Thermal/ECS/Turbine  press_Turbine_exit=80  inertia=5e-5  n_t=0.7
  User-set_ supply_pressure : Subsystem
  Valve1 : Subsystem
  valve  opening : Integrator  InitialCondition=.4  LimitOutput=on  UpperSaturationLimit=.8  LowerSaturationLimit=.2
  valve  opening1 : Integrator  InitialCondition=.5  LimitOutput=on  UpperSaturationLimit=1  LowerSaturationLimit=.3
  Reqd. Bleed air : Outport
  Flow Out : Outport  Port=2
  wires:
  Constant1/1 -> Sum1/1
  PID Controller1/1 -> [bleed_valve], Scope1/1  "Bleed air to valve"
  Sum1/1 -> PID Controller1/1
  Bus Selector3/1 -> Sum1/2  "<temp_K>"
  [pHX_in] -> Primary HX (air-air)/1
  Valve1/1(Flow Out) -> Mixing Junction/1
  [Flow_to_valve] -> Valve1/1(Flow In)
  [Shaft_speed] -> Compressor/2
  Compressor/2 -> Turbine/2
  Ram air inlet/1(Flow Out) -> Primary HX (air-air)/2, [ram_air]
  Compressor/1 -> Secondary  HX (air-air)/1
  [ram_air] -> Secondary  HX (air-air)/2
  Mixing Junction/1 -> User-set_ supply_pressure/1(Flow In)
  Turbine/2 -> [Shaft_speed]
  Turbine/3 -> Terminator1/1
  Turbine/1 -> [turb_out]
  User-set_ supply_pressure/1(Flow Out) -> Flow Out/1
  [Cabin_pressure] -> User-set_ supply_pressure/2(Cabin Pres.)  "pres_kPa"
  [temp_amb_K] -> Ram air inlet/1(Temp_amb)
  [pHX_out] -> Ram air inlet/2(Temp_comp)
  MISSION/1 -> Bus Selector/1
  CONTROL/1 -> Terminator2/1
  ENGINE/1 -> Bus Selector4/1
  Distribution of bleed air/2(Flow to HX) -> [pHX_in]
  Distribution of bleed air/1(Flow to Mix Junc.) -> [Flow_to_valve]
  Bus Selector4/1 -> Gain2/1  "<BleedAirTemp_K>"
  Bus Selector4/2 -> Gain3/1  "<BleedAirPres_kPa>"
  Bus Selector/2 -> [temp_amb_K]  "<temp_K>"
  Bus Selector/1 -> [Mach_number]  "<Mach>"
  Gain1/1 -> Distribution of bleed air/1(Bleed to Valve), Sum2/1  "mdot_kgps"
  Gain2/1 -> Distribution of bleed air/3(bleed_temp)  "temp_K"
  Gain3/1 -> Distribution of bleed air/4(bleed_pres)  "pres_kPa"
  [bleed_valve] -> Gain1/1
  Primary HX (air-air)/3 -> Terminator3/1
  Primary HX (air-air)/2 -> Terminator/1
  Primary HX (air-air)/1 -> [pHX_out]
  Secondary  HX (air-air)/2 -> Terminator5/1
  Secondary  HX (air-air)/3 -> Terminator7/1
  Secondary  HX (air-air)/1 -> Turbine/1
  [pHX_out] -> Subsystem1/2(Air from PHX)
  Mixing Junction2/1 -> [junc273], Mixing Junction/2
  [turb_out] -> Mixing Junction2/1
  Subsystem1/1(Air to Mix Junc) -> Mixing Junction2/2
  Subsystem1/2(Air to Comp) -> Compressor/1
  [junc273] -> Bus Selector1/1
  Bus Selector1/1 -> Sum/2  "<temp_K>"
  Sum/1 -> PID Controller/1, Scope4/1
  PID Controller/1 -> valve  opening/1
  valve  opening/1 -> Scope3/1, [bleed_acm]  "Valve Opening"
  Constant/1 -> Sum/1
  Gain4/1 -> Distribution of bleed air/2(Bleed to ACM), Sum2/2  "mdot_kgps"
  Sum2/1 -> Reqd. Bleed air/1
  [turb_out] -> Bus Selector2/1
  Bus Selector2/1 -> Sum3/2  "<temp_K>"
  Sum3/1 -> PID Controller2/1, Scope2/1
  PID Controller2/1 -> valve  opening1/1  "Valve Opening"
  Constant3/1 -> Sum3/1
  valve  opening1/1 -> Scope/1  "Valve Opening"
  Cabin Conditions/1 -> Bus Selector3/1
  [bleed_acm] -> Gain4/1
  Constant2/1 -> Subsystem1/1(Bypass Ratio)

== system Boeing737Sample_updatedCopy/ECS & FOS /Oil Tanks/Pumps Left Wing ==
  Oil Sys Pres : Inport
  Flow In : Inport  Port=2
  Bus Selector1 : BusSelector  OutputSignals=Oil
  Bus Selector2 : BusSelector  OutputSignals=real_pwr_W,react_pwr_VAr
  Bus Selector5 : BusSelector  OutputSignals=mdot_kgps,pres_kPa
  ElectricalSink1 : PowerFlowLib/Support Functions//Tools/ElectricalSink  Tag=Flow  Description=TwoPhase  load_loc=LeftWing  ACDC_load=AC  units=Watts  unq_id=1878
  Fuel Switch2 : Constant  Value=1400
  Ground : Ground
  Ground1 : Ground
  Oil Pump : PowerFlowLib/Energy & Power Systems/Thermal/Oil/Oil Pump  maptype=Pressure (kPa) vs. Vol. Flow Rate (m³/hr)  map=B737_mech_fuel1  map_load=off  SG=0.82  pump_eff=.75  heat_out=off  AC_pwr=on  pf=1  mech_pwr=off
  Oil Tank : PowerFlowLib/Energy & Power Systems/Thermal/Fuel/Fuel Tank  fileslct=off  filename=fueltank_area.m  filedir=C:\Users\mwillms4\Documents\My Box Files\Graduate\Research\PowerFlow Development\PowerFlow Fall 2013\SupportFunctions\fueltank_area.m  tank_loc=Left Wing Tank  areaprompt2=off  max_vol=3.2  m_init=2500  fld_Tint=0  ull_Tint=30  Pover=100  HTC_fg=14.2  wallHXF=off  wetHTC=14.2  dryHTC=14.2  Qinternal=0
  Terminator : Terminator
  Terminator1 : Terminator
  Oil To HX : Outport
  wires:
  Bus Selector5/1 -> Oil Tank/2  "<mdot_kgps>"
  Fuel Switch2/1 -> Oil Pump/2
  Flow In/1 -> Bus Selector1/1
  Oil Sys Pres/1 -> Oil Pump/3
  Ground1/1 -> Oil Tank/3
  Oil Pump/1 -> Oil To HX/1, Bus Selector5/1
  Oil Pump/3 -> Oil Tank/4
  Ground/1 -> Oil Tank/5
  Oil Tank/3 -> Terminator1/1
  Oil Tank/2 -> Terminator/1
  Oil Tank/1 -> Oil Pump/1
  Bus Selector2/1 -> ElectricalSink1/1  "<real_pwr_W>"
  Bus Selector2/2 -> ElectricalSink1/2  "<react_pwr_VAr>"
  Oil Pump/2 -> Bus Selector2/1
  Bus Selector1/1 -> Oil Tank/1  "<Oil>"

== system Boeing737Sample_updatedCopy/ECS & FOS /Oil Tanks/Pumps Right Wing ==
  Oil Sys Pres : Inport
  Flow In : Inport  Port=2
  Bus Selector1 : BusSelector  OutputSignals=Oil
  Bus Selector2 : BusSelector  OutputSignals=real_pwr_W,react_pwr_VAr
  Bus Selector5 : BusSelector  OutputSignals=mdot_kgps,pres_kPa
  ElectricalSink1 : PowerFlowLib/Support Functions//Tools/ElectricalSink  Tag=Flow  Description=TwoPhase  load_loc=RightWing  ACDC_load=AC  units=Watts  unq_id=3506
  Fuel Switch2 : Constant  Value=1400
  Fuel Tank : PowerFlowLib/Energy & Power Systems/Thermal/Fuel/Fuel Tank  fileslct=off  filename=fueltank_area.m  filedir=C:\Users\mwillms4\Documents\My Box Files\Graduate\Research\PowerFlow Development\PowerFlow Fall 2013\SupportFunctions\fueltank_area.m  tank_loc=Left Wing Tank  areaprompt2=off  max_vol=3.2  m_init=2500  fld_Tint=0  ull_Tint=30  Pover=100  HTC_fg=14.2  wallHXF=off  wetHTC=14.2  dryHTC=14.2  Qinternal=0
  Ground : Ground
  Ground1 : Ground
  Oil Pump : PowerFlowLib/Energy & Power Systems/Thermal/Oil/Oil Pump  maptype=Pressure (kPa) vs. Vol. Flow Rate (m³/hr)  map=B737_mech_fuel1  map_load=off  SG=0.82  pump_eff=.75  heat_out=off  AC_pwr=on  pf=1  mech_pwr=off
  Terminator : Terminator
  Terminator1 : Terminator
  Oil To HX : Outport
  wires:
  Fuel Tank/1 -> Oil Pump/1
  Fuel Tank/2 -> Terminator/1
  Fuel Tank/3 -> Terminator1/1
  Ground/1 -> Fuel Tank/5
  Oil Pump/3 -> Fuel Tank/4
  Oil Pump/1 -> Bus Selector5/1, Oil To HX/1
  Ground1/1 -> Fuel Tank/3
  Oil Sys Pres/1 -> Oil Pump/3
  Flow In/1 -> Bus Selector1/1
  Fuel Switch2/1 -> Oil Pump/2
  Bus Selector5/1 -> Fuel Tank/2  "<mdot_kgps>"
  Bus Selector2/1 -> ElectricalSink1/1  "<real_pwr_W>"
  Bus Selector2/2 -> ElectricalSink1/2  "<react_pwr_VAr>"
  Oil Pump/2 -> Bus Selector2/1
  Bus Selector1/1 -> Fuel Tank/1  "<Oil>"

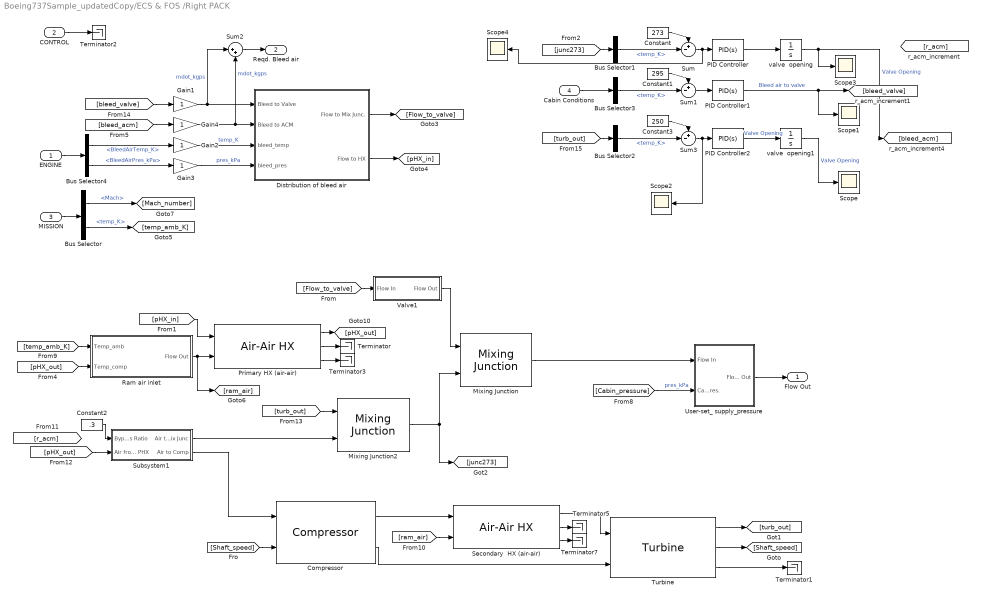
== system Boeing737Sample_updatedCopy/ECS & FOS /Right PACK ==
  ENGINE : Inport
  CONTROL : Inport  Port=2
  MISSION : Inport  Port=3
  Cabin Conditions : Inport  Port=4
  Bus Selector : BusSelector  OutputSignals=Flight parameters.Mach,Flight parameters.temp_K
  Bus Selector1 : BusSelector  OutputSignals=temp_K
  Bus Selector2 : BusSelector  OutputSignals=temp_K
  Bus Selector3 : BusSelector  OutputSignals=temp_K
  Bus Selector4 : BusSelector  OutputSignals=Bleed.BleedAirTemp_K,Bleed.BleedAirPres_kPa
  Compressor : PowerFlowLib/Energy & Power Systems/Thermal/ECS/Compressor
  Constant : Constant  Value=273
  Constant1 : Constant  Value=295
  Constant2 : Constant  Value=.3
  Constant3 : Constant  Value=250
  Distribution of bleed air : Subsystem
      mask Display:
      | port_label('input',1,'{ \bfBleed air to valve [kg/s]}','texmode','on')
      | port_label('input',2,'{ \bfBleed air to ACM [kg/s]}','texmode','on')
      | port_label('input',3,'{ \bfBleed temp. (K)}','texmode','on');
      | port_label('input',4,'{ \bfBleed pressure. (kPa)}','texmode','on')
      | 
      | 
      | 
      | port_label('output',1,'{\bfFlow to Mix Junc. }','texmode','on')
      | port_label('output',2,'{\bfFlow to ACM }','texmode','on')
  Gain{1..4} (4 alike) : Gain
  Mixing Junction : PowerFlowLib/Energy & Power Systems/Thermal/ECS/Mixing Junction  d_in_1=0.1  d_in_2=0.1  d_out=0.2
  Mixing Junction2 : PowerFlowLib/Energy & Power Systems/Thermal/ECS/Mixing Junction  d_in_1=0.1  d_in_2=0.1  d_out=0.2
  PID Controller : simulink/Continuous/PID Controller  Controller=PID  TimeDomain=Continuous-time  SampleTime=1  IntegratorMethod=Forward Euler  FilterMethod=Forward Euler  Form=Parallel  P=.01  I=0  D=0  N=100  InitialConditionSource=internal  InitialConditionForIntegrator=0  InitialConditionForFilter=0  ExternalReset=none  LimitOutput=off  UpperSaturationLimit=inf  LowerSaturationLimit=-inf  LinearizeAsGain=off  AntiWindupMode=none  Kb=1  TrackingMode=off  Kt=1  PParamMin=[]  PParamMax=[]  IParamMin=[]  IParamMax=[]  DParamMin=[]  DParamMax=[]  NParamMin=[]  NParamMax=[]  KbParamMin=[]  KbParamMax=[]  KtParamMin=[]  KtParamMax=[]  POutMin=[]  POutMax=[]  IOutMin=[]  IOutMax=[]  DOutMin=[]  DOutMax=[]  NOutMin=[]  NOutMax=[]  KbOutMin=[]  KbOutMax=[]  KtOutMin=[]  KtOutMax=[]  IntegratorOutMin=[]  IntegratorOutMax=[]  FilterOutMin=[]  FilterOutMax=[]  SumOutMin=[]  SumOutMax=[]  SumI1OutMin=[]  SumI1OutMax=[]  SumI2OutMin=[]  SumI2OutMax=[]  SumI3OutMin=[]  SumI3OutMax=[]  SumDOutMin=[]  SumDOutMax=[]  SaturationOutMin=[]  SaturationOutMax=[]  IntegratorContinuousStateAttributes=''  IntegratorStateMustResolveToSignalObject=off  IntegratorRTWStateStorageClass=Auto  FilterContinuousStateAttributes=''  FilterStateMustResolveToSignalObject=off  FilterRTWStateStorageClass=Auto
  PID Controller1 : simulink/Continuous/PID Controller  Controller=PID  TimeDomain=Continuous-time  SampleTime=1  IntegratorMethod=Forward Euler  FilterMethod=Forward Euler  Form=Parallel  P=.2  I=.01  D=0  N=100  InitialConditionSource=internal  InitialConditionForIntegrator=0  InitialConditionForFilter=0  ExternalReset=none  LimitOutput=on  UpperSaturationLimit=2  LowerSaturationLimit=.05  LinearizeAsGain=off  AntiWindupMode=none  Kb=1  TrackingMode=off  Kt=1  PParamMin=[]  PParamMax=[]  IParamMin=[]  IParamMax=[]  DParamMin=[]  DParamMax=[]  NParamMin=[]  NParamMax=[]  KbParamMin=[]  KbParamMax=[]  KtParamMin=[]  KtParamMax=[]  POutMin=[]  POutMax=[]  IOutMin=[]  IOutMax=[]  DOutMin=[]  DOutMax=[]  NOutMin=[]  NOutMax=[]  KbOutMin=[]  KbOutMax=[]  KtOutMin=[]  KtOutMax=[]  IntegratorOutMin=[]  IntegratorOutMax=[]  FilterOutMin=[]  FilterOutMax=[]  SumOutMin=[]  SumOutMax=[]  SumI1OutMin=[]  SumI1OutMax=[]  SumI2OutMin=[]  SumI2OutMax=[]  SumI3OutMin=[]  SumI3OutMax=[]  SumDOutMin=[]  SumDOutMax=[]  SaturationOutMin=[]  SaturationOutMax=[]  IntegratorContinuousStateAttributes=''  IntegratorStateMustResolveToSignalObject=off  IntegratorRTWStateStorageClass=Auto  FilterContinuousStateAttributes=''  FilterStateMustResolveToSignalObject=off  FilterRTWStateStorageClass=Auto
  PID Controller2 : simulink/Continuous/PID Controller  Controller=PID  TimeDomain=Continuous-time  SampleTime=1  IntegratorMethod=Forward Euler  FilterMethod=Forward Euler  Form=Parallel  P=0.01  I=0  D=0  N=100  InitialConditionSource=internal  InitialConditionForIntegrator=0  InitialConditionForFilter=0  ExternalReset=none  LimitOutput=off  UpperSaturationLimit=inf  LowerSaturationLimit=0  LinearizeAsGain=off  AntiWindupMode=none  Kb=1  TrackingMode=off  Kt=1  PParamMin=[]  PParamMax=[]  IParamMin=[]  IParamMax=[]  DParamMin=[]  DParamMax=[]  NParamMin=[]  NParamMax=[]  KbParamMin=[]  KbParamMax=[]  KtParamMin=[]  KtParamMax=[]  POutMin=[]  POutMax=[]  IOutMin=[]  IOutMax=[]  DOutMin=[]  DOutMax=[]  NOutMin=[]  NOutMax=[]  KbOutMin=[]  KbOutMax=[]  KtOutMin=[]  KtOutMax=[]  IntegratorOutMin=[]  IntegratorOutMax=[]  FilterOutMin=[]  FilterOutMax=[]  SumOutMin=[]  SumOutMax=[]  SumI1OutMin=[]  SumI1OutMax=[]  SumI2OutMin=[]  SumI2OutMax=[]  SumI3OutMin=[]  SumI3OutMax=[]  SumDOutMin=[]  SumDOutMax=[]  SaturationOutMin=[]  SaturationOutMax=[]  IntegratorContinuousStateAttributes=''  IntegratorStateMustResolveToSignalObject=off  IntegratorRTWStateStorageClass=Auto  FilterContinuousStateAttributes=''  FilterStateMustResolveToSignalObject=off  FilterRTWStateStorageClass=Auto
  Primary HX (air-air) : PowerFlowLib/Energy & Power Systems/Thermal/ECS/Air-Air HX  L_hx=0.2  W_hx=0.2  H_hx=0.2  t_p=0.0008  K_p=167  cp_hx=883  m_cm=16  l_fin=.005  t_fin=0.0002  s_fin=0.0015  h_fin=0.0095  K_n=167  eta_f=0.8  T_cm_0=50
  Ram air inlet : Subsystem  mask{ram_air=.5, T_35=273}
      mask prompts: ram_air "Ram air mass flow rate"; T_35 "Temperature control for 35F valve"
      mask Display:
      | port_label('input',1,'{ \bf Ambient Temp.}','texmode','on')
      | port_label('input',2,'{ \bf Comp. Face Temp.}','texmode','on');
      | 
      | port_label('output',1,'{\bf Flow Out}','texmode','on')
  Scope{,1..4} (5 alike) : Scope
      Scope settings: SaveName=ScopeData32  SampleInput=on  SampleTime=1
      Scope1 settings: YMin=0  YMax=0.375  SaveName=ScopeData33  SampleInput=on  SampleTime=1
      Scope2 settings: YMin=-0.07  YMax=-0.0325  SaveName=ScopeData34  SampleInput=on  SampleTime=1
      Scope3 settings: YMin=0.427  YMax=0.437  SaveName=ScopeData35  SampleInput=on  SampleTime=1
      Scope4 settings: YMin=0.048825  YMax=0.04905  SaveName=ScopeData37  SampleInput=on  SampleTime=1
  Secondary  HX (air-air) : PowerFlowLib/Energy & Power Systems/Thermal/ECS/Air-Air HX  L_hx=0.2  W_hx=0.2  H_hx=0.2  t_p=0.0008  K_p=167  cp_hx=883  m_cm=16  l_fin=.005  t_fin=0.0002  s_fin=0.0015  h_fin=0.0095  K_n=167  eta_f=0.8  T_cm_0=25
  Subsystem1 : Subsystem
  Sum : Sum  Inputs=+-|
  Sum1 : Sum  Inputs=+-|
  Sum2 : Sum  Inputs=|++
  Sum3 : Sum  Inputs=+-|
  Terminator{,1..3,5,7} (6 alike) : Terminator
  Turbine : PowerFlowLib/Energy & Power Systems/Thermal/ECS/Turbine  press_Turbine_exit=80  inertia=5e-5  n_t=0.7
  User-set_ supply_pressure : Subsystem
  Valve1 : Subsystem
  valve  opening : Integrator  InitialCondition=.5  LimitOutput=on  UpperSaturationLimit=0.8  LowerSaturationLimit=0.2
  valve  opening1 : Integrator  InitialCondition=.5  LimitOutput=on  UpperSaturationLimit=1  LowerSaturationLimit=.3
  Flow Out : Outport
  Reqd. Bleed air : Outport  Port=2
  wires:
  Cabin Conditions/1 -> Bus Selector3/1
  valve  opening1/1 -> Scope/1  "Valve Opening"
  Constant3/1 -> Sum3/1
  PID Controller2/1 -> valve  opening1/1  "Valve Opening"
  Sum3/1 -> Scope2/1, PID Controller2/1
  Bus Selector2/1 -> Sum3/2  "<temp_K>"
  [turb_out] -> Bus Selector2/1
  Sum2/1 -> Reqd. Bleed air/1
  Gain4/1 -> Sum2/2, Distribution of bleed air/2(Bleed to ACM)  "mdot_kgps"
  Constant/1 -> Sum/1
  valve  opening/1 -> Scope3/1, [bleed_acm]  "Valve Opening"
  PID Controller/1 -> valve  opening/1
  Sum/1 -> Scope4/1, PID Controller/1
  Bus Selector1/1 -> Sum/2  "<temp_K>"
  [junc273] -> Bus Selector1/1
  Subsystem1/2(Air to Comp) -> Compressor/1
  Subsystem1/1(Air to Mix Junc) -> Mixing Junction2/2
  [turb_out] -> Mixing Junction2/1
  Mixing Junction2/1 -> Mixing Junction/2, [junc273]
  [pHX_out] -> Subsystem1/2(Air from PHX)
  Secondary  HX (air-air)/1 -> Turbine/1
  Secondary  HX (air-air)/3 -> Terminator7/1
  Secondary  HX (air-air)/2 -> Terminator5/1
  Primary HX (air-air)/1 -> [pHX_out]
  Primary HX (air-air)/2 -> Terminator/1
  Primary HX (air-air)/3 -> Terminator3/1
  [bleed_valve] -> Gain1/1
  Gain3/1 -> Distribution of bleed air/4(bleed_pres)  "pres_kPa"
  Gain2/1 -> Distribution of bleed air/3(bleed_temp)  "temp_K"
  Gain1/1 -> Sum2/1, Distribution of bleed air/1(Bleed to Valve)  "mdot_kgps"
  Bus Selector/1 -> [Mach_number]  "<Mach>"
  Bus Selector/2 -> [temp_amb_K]  "<temp_K>"
  Bus Selector4/2 -> Gain3/1  "<BleedAirPres_kPa>"
  Bus Selector4/1 -> Gain2/1  "<BleedAirTemp_K>"
  Distribution of bleed air/1(Flow to Mix Junc.) -> [Flow_to_valve]
  Distribution of bleed air/2(Flow to HX) -> [pHX_in]
  ENGINE/1 -> Bus Selector4/1
  CONTROL/1 -> Terminator2/1
  MISSION/1 -> Bus Selector/1
  [pHX_out] -> Ram air inlet/2(Temp_comp)
  [temp_amb_K] -> Ram air inlet/1(Temp_amb)
  [Cabin_pressure] -> User-set_ supply_pressure/2(Cabin Pres.)  "pres_kPa"
  User-set_ supply_pressure/1(Flow Out) -> Flow Out/1
  Turbine/1 -> [turb_out]
  Turbine/3 -> Terminator1/1
  Turbine/2 -> [Shaft_speed]
  Mixing Junction/1 -> User-set_ supply_pressure/1(Flow In)
  [ram_air] -> Secondary  HX (air-air)/2
  Compressor/1 -> Secondary  HX (air-air)/1
  Ram air inlet/1(Flow Out) -> [ram_air], Primary HX (air-air)/2
  Compressor/2 -> Turbine/2
  [Shaft_speed] -> Compressor/2
  [Flow_to_valve] -> Valve1/1(Flow In)
  Valve1/1(Flow Out) -> Mixing Junction/1
  [pHX_in] -> Primary HX (air-air)/1
  Bus Selector3/1 -> Sum1/2  "<temp_K>"
  Sum1/1 -> PID Controller1/1
  PID Controller1/1 -> Scope1/1, [bleed_valve]  "Bleed air to valve"
  Constant1/1 -> Sum1/1
  [bleed_acm] -> Gain4/1
  Constant2/1 -> Subsystem1/1(Bypass Ratio)
